simulink model "FaultFeeder"  (R2019a)
settings: Solver=ode1  StartTime=0.0  StopTime=2.5  FixedStep=Ts_Power  RelTol=1e-3
PostLoadFcn:
  | %% Init for wind PnO models - global system parameters
  | OVERRIDE_SSN_MEMORY_LIMIT=1;
  | Ts=50e-6;
  | % Ts=50e-10;
  | Ts_Power=Ts;
  | Ts_Control=2*Ts;
  | freq = 50;
  | Fnom=freq;
  | Vac=400e3;
InitFcn:
  | %% Init for wind PnO models - global system parameters
  | OVERRIDE_SSN_MEMORY_LIMIT=1;
  | Ts=50e-6;
  | % Ts=50e-10;
  | Ts_Power=Ts;
  | Ts_Control=2*Ts;
  | freq = 50;
  | Fnom=freq;
  | Vac=225e3;
values from neighbouring files (symbols this model uses):
  feeder_posCap = 0.2e-006    (= 2e-07)    [variable.m]
  feeder_posInd = 0.00040107    [variable.m]
  feeder_posR = 0.14    [variable.m]
  feeder_zeroCap = 0.08    [variable.m]
  feeder_zeroInd = 0.00120321    [variable.m]
  feeder_zeroR = 0.42    [variable.m]
  sub_posCap = 0.16e-006    (= 1.6e-07)    [variable.m]
  sub_posInd = 0.001400563    [variable.m]
  sub_posR = 0.036    [variable.m]
  sub_zeroCap = 0.053333e-006    (= 5.3333e-08)    [variable.m]
  sub_zeroInd = 0.00420169    [variable.m]
  sub_zeroR = 0.108    [variable.m]
  transfo_L1 = 0.05999374    [variable.m]
  transfo_L2 = 0.05999374    [variable.m]
  transfo_R1 = 0.000866667    [variable.m]
  transfo_R2 = 0.00086667    [variable.m]
undefined symbols (not defined in the file or in its folder): D1, D11, Delta, den, DiscIntNeverNeededParam, dx, find_system, gcbh, num, out_Buses, out_WindFarms, sps_rtmsupport
libraries: powerlib x196, simulink x96, powerlib_meascontrol x96, elements x52, eeSinusoidalMeasurement x49, simulink_extras x42, spsVIMeasurementModel x33, eePowerMeasurement x15
(part 22 of 24)

== system FaultFeeder/SM_WT1/Wind Type IV Detailed v2.1 - 4/Control/Measurement and Transformation/Discrete 3-phase PLL-Driven Positive-Sequence Active & Reactive Power/Discrete 3-phase PLL-Driven Positive-Sequence Fundamental Value2 ==
  note: Discrete 3-phase PLL-Driven Positive-Sequence Fundamental Value
  note: Pierre Giroux, Gilbert Sybille
      | Power System Simulation Laboratory
      | IREQ, Hydro-Quebc
  Freq : Inport
  w : Inport  Port=2  PortDimensions=1
  abc : Inport  Port=3  PortDimensions=3
  Cartesian to Polar : simulink_extras/Transformations/Cartesian to Polar
  Demux : Demux  Outputs=3
  Discrete Variable Frequency Mean value1 : Subsystem  mask(Discrete Variable-Frequency Mean Value){Finit=Finit, Fmin=Fmin, Vinit=Imag_Init, Ts=Ts}
      mask prompts: Finit "Initial frequency (Hz):"; Fmin "Minimum frequency (Hz):"; Vinit "Initial input (DC component):"; Ts "Sample time:"
      mask help:
      | This discrete block computes the mean value of the input signal (port In) over a running window of one cycle of a specified frequency (port Freq).
      |
      | For the first cycle of simulation (specified by the parameter "Initial frequency"), the output is held to the value of the  "Initial input" parameter.
      |
      | The value of the parameter "Minimum frequency" is used to determine the buffer size of the "Variable Transport Delay" block found inside this subsystem.
      mask init:
      | MaxDelay=1/Fmin+Ts;
      | power_initmask();
      settings: OpenFcn=power_openblockproxy();
  Discrete Variable Frequency Mean value2 : Subsystem  mask(Discrete Variable-Frequency Mean Value){Finit=Finit, Fmin=Fmin, Vinit=Real_Init, Ts=Ts}
      mask prompts: Finit "Initial frequency (Hz):"; Fmin "Minimum frequency (Hz):"; Vinit "Initial input (DC component):"; Ts "Sample time:"
      mask help:
      | This discrete block computes the mean value of the input signal (port In) over a running window of one cycle of a specified frequency (port Freq).
      |
      | For the first cycle of simulation (specified by the parameter "Initial frequency"), the output is held to the value of the  "Initial input" parameter.
      |
      | The value of the parameter "Minimum frequency" is used to determine the buffer size of the "Variable Transport Delay" block found inside this subsystem.
      mask init:
      | MaxDelay=1/Fmin+Ts;
      | power_initmask();
      settings: OpenFcn=power_openblockproxy();
  Rad->Deg. : Gain  Gain=180/pi  SaturateOnIntegerOverflow=on  OutDataTypeStr=Inherit: Same as input  ParamDataTypeStr=Inherit: Same as input
  Terminator : Terminator
  abc to dq0 : powerlib_meascontrol/Transformations/abc to dq0  Alignment=90 degrees behind phase A axis
  Mag : Outport  VectorParamsAs1DForOutWhenUnconnected=on
  Phase : Outport  Port=2  VectorParamsAs1DForOutWhenUnconnected=on
  wires:
  Cartesian to Polar/2 -> Rad->Deg./1
  Cartesian to Polar/1 -> Mag/1
  Demux/3 -> Terminator/1
  abc to dq0/1 -> Demux/1
  abc/1 -> abc to dq0/1
  Demux/1 -> Discrete Variable Frequency Mean value2/2(In)
  Demux/2 -> Discrete Variable Frequency Mean value1/2(In)
  Discrete Variable Frequency Mean value1/1(Mean) -> Cartesian to Polar/2  "Real"
  Rad->Deg./1 -> Phase/1
  Discrete Variable Frequency Mean value2/1(Mean) -> Cartesian to Polar/1  "Real"
  Freq/1 -> Discrete Variable Frequency Mean value1/1(Freq), Discrete Variable Frequency Mean value2/1(Freq)
  w/1 -> abc to dq0/2

== system FaultFeeder/SM_WT1/Wind Type IV Detailed v2.1 - 5/Control/Measurement and Transformation/Discrete 3-phase PLL-Driven Positive-Sequence Active & Reactive Power/Discrete 3-phase PLL-Driven Positive-Sequence Fundamental Value ==
  note: Pierre Giroux, Gilbert Sybille
      | Power System Simulation Laboratory
      | IREQ, Hydro-Quebc
  note: Discrete 3-phase PLL-Driven Positive-Sequence Fundamental Value
  Freq : Inport
  w : Inport  Port=2  PortDimensions=1
  abc : Inport  Port=3  PortDimensions=3
  Cartesian to Polar : simulink_extras/Transformations/Cartesian to Polar
  Demux : Demux  Outputs=3
  Discrete Variable Frequency Mean value1 : Subsystem  mask(Discrete Variable-Frequency Mean Value){Finit=Finit, Fmin=Fmin, Vinit=Imag_Init, Ts=Ts}
      mask prompts: Finit "Initial frequency (Hz):"; Fmin "Minimum frequency (Hz):"; Vinit "Initial input (DC component):"; Ts "Sample time:"
      mask help:
      | This discrete block computes the mean value of the input signal (port In) over a running window of one cycle of a specified frequency (port Freq).
      |
      | For the first cycle of simulation (specified by the parameter "Initial frequency"), the output is held to the value of the  "Initial input" parameter.
      |
      | The value of the parameter "Minimum frequency" is used to determine the buffer size of the "Variable Transport Delay" block found inside this subsystem.
      mask init:
      | MaxDelay=1/Fmin+Ts;
      | power_initmask();
      settings: OpenFcn=power_openblockproxy();
  Discrete Variable Frequency Mean value2 : Subsystem  mask(Discrete Variable-Frequency Mean Value){Finit=Finit, Fmin=Fmin, Vinit=Real_Init, Ts=Ts}
      mask prompts: Finit "Initial frequency (Hz):"; Fmin "Minimum frequency (Hz):"; Vinit "Initial input (DC component):"; Ts "Sample time:"
      mask help:
      | This discrete block computes the mean value of the input signal (port In) over a running window of one cycle of a specified frequency (port Freq).
      |
      | For the first cycle of simulation (specified by the parameter "Initial frequency"), the output is held to the value of the  "Initial input" parameter.
      |
      | The value of the parameter "Minimum frequency" is used to determine the buffer size of the "Variable Transport Delay" block found inside this subsystem.
      mask init:
      | MaxDelay=1/Fmin+Ts;
      | power_initmask();
      settings: OpenFcn=power_openblockproxy();
  Rad->Deg. : Gain  Gain=180/pi  SaturateOnIntegerOverflow=on  OutDataTypeStr=Inherit: Same as input  ParamDataTypeStr=Inherit: Same as input
  Terminator : Terminator
  abc to dq0 : powerlib_meascontrol/Transformations/abc to dq0  Alignment=90 degrees behind phase A axis
  Mag : Outport  VectorParamsAs1DForOutWhenUnconnected=on
  Phase : Outport  Port=2  VectorParamsAs1DForOutWhenUnconnected=on
  wires:
  w/1 -> abc to dq0/2
  Freq/1 -> Discrete Variable Frequency Mean value2/1(Freq), Discrete Variable Frequency Mean value1/1(Freq)
  Discrete Variable Frequency Mean value2/1(Mean) -> Cartesian to Polar/1  "Real"
  Rad->Deg./1 -> Phase/1
  Discrete Variable Frequency Mean value1/1(Mean) -> Cartesian to Polar/2  "Real"
  Demux/2 -> Discrete Variable Frequency Mean value1/2(In)
  Demux/1 -> Discrete Variable Frequency Mean value2/2(In)
  abc/1 -> abc to dq0/1
  abc to dq0/1 -> Demux/1
  Demux/3 -> Terminator/1
  Cartesian to Polar/1 -> Mag/1
  Cartesian to Polar/2 -> Rad->Deg./1

== system FaultFeeder/SM_WT1/Wind Type IV Detailed v2.1 - 5/Control/Measurement and Transformation/Discrete 3-phase PLL-Driven Positive-Sequence Active & Reactive Power/Discrete 3-phase PLL-Driven Positive-Sequence Fundamental Value2 ==
  note: Discrete 3-phase PLL-Driven Positive-Sequence Fundamental Value
  note: Pierre Giroux, Gilbert Sybille
      | Power System Simulation Laboratory
      | IREQ, Hydro-Quebc
  Freq : Inport
  w : Inport  Port=2  PortDimensions=1
  abc : Inport  Port=3  PortDimensions=3
  Cartesian to Polar : simulink_extras/Transformations/Cartesian to Polar
  Demux : Demux  Outputs=3
  Discrete Variable Frequency Mean value1 : Subsystem  mask(Discrete Variable-Frequency Mean Value){Finit=Finit, Fmin=Fmin, Vinit=Imag_Init, Ts=Ts}
      mask prompts: Finit "Initial frequency (Hz):"; Fmin "Minimum frequency (Hz):"; Vinit "Initial input (DC component):"; Ts "Sample time:"
      mask help:
      | This discrete block computes the mean value of the input signal (port In) over a running window of one cycle of a specified frequency (port Freq).
      |
      | For the first cycle of simulation (specified by the parameter "Initial frequency"), the output is held to the value of the  "Initial input" parameter.
      |
      | The value of the parameter "Minimum frequency" is used to determine the buffer size of the "Variable Transport Delay" block found inside this subsystem.
      mask init:
      | MaxDelay=1/Fmin+Ts;
      | power_initmask();
      settings: OpenFcn=power_openblockproxy();
  Discrete Variable Frequency Mean value2 : Subsystem  mask(Discrete Variable-Frequency Mean Value){Finit=Finit, Fmin=Fmin, Vinit=Real_Init, Ts=Ts}
      mask prompts: Finit "Initial frequency (Hz):"; Fmin "Minimum frequency (Hz):"; Vinit "Initial input (DC component):"; Ts "Sample time:"
      mask help:
      | This discrete block computes the mean value of the input signal (port In) over a running window of one cycle of a specified frequency (port Freq).
      |
      | For the first cycle of simulation (specified by the parameter "Initial frequency"), the output is held to the value of the  "Initial input" parameter.
      |
      | The value of the parameter "Minimum frequency" is used to determine the buffer size of the "Variable Transport Delay" block found inside this subsystem.
      mask init:
      | MaxDelay=1/Fmin+Ts;
      | power_initmask();
      settings: OpenFcn=power_openblockproxy();
  Rad->Deg. : Gain  Gain=180/pi  SaturateOnIntegerOverflow=on  OutDataTypeStr=Inherit: Same as input  ParamDataTypeStr=Inherit: Same as input
  Terminator : Terminator
  abc to dq0 : powerlib_meascontrol/Transformations/abc to dq0  Alignment=90 degrees behind phase A axis
  Mag : Outport  VectorParamsAs1DForOutWhenUnconnected=on
  Phase : Outport  Port=2  VectorParamsAs1DForOutWhenUnconnected=on
  wires:
  Cartesian to Polar/2 -> Rad->Deg./1
  Cartesian to Polar/1 -> Mag/1
  Demux/3 -> Terminator/1
  abc to dq0/1 -> Demux/1
  abc/1 -> abc to dq0/1
  Demux/1 -> Discrete Variable Frequency Mean value2/2(In)
  Demux/2 -> Discrete Variable Frequency Mean value1/2(In)
  Discrete Variable Frequency Mean value1/1(Mean) -> Cartesian to Polar/2  "Real"
  Rad->Deg./1 -> Phase/1
  Discrete Variable Frequency Mean value2/1(Mean) -> Cartesian to Polar/1  "Real"
  Freq/1 -> Discrete Variable Frequency Mean value1/1(Freq), Discrete Variable Frequency Mean value2/1(Freq)
  w/1 -> abc to dq0/2

== system FaultFeeder/SM_WT1/Wind Type IV Detailed v2.1 - 6/Control/Measurement and Transformation/Discrete 3-phase PLL-Driven Positive-Sequence Active & Reactive Power/Discrete 3-phase PLL-Driven Positive-Sequence Fundamental Value ==
  note: Pierre Giroux, Gilbert Sybille
      | Power System Simulation Laboratory
      | IREQ, Hydro-Quebc
  note: Discrete 3-phase PLL-Driven Positive-Sequence Fundamental Value
  Freq : Inport
  w : Inport  Port=2  PortDimensions=1
  abc : Inport  Port=3  PortDimensions=3
  Cartesian to Polar : simulink_extras/Transformations/Cartesian to Polar
  Demux : Demux  Outputs=3
  Discrete Variable Frequency Mean value1 : Subsystem  mask(Discrete Variable-Frequency Mean Value){Finit=Finit, Fmin=Fmin, Vinit=Imag_Init, Ts=Ts}
      mask prompts: Finit "Initial frequency (Hz):"; Fmin "Minimum frequency (Hz):"; Vinit "Initial input (DC component):"; Ts "Sample time:"
      mask help:
      | This discrete block computes the mean value of the input signal (port In) over a running window of one cycle of a specified frequency (port Freq).
      |
      | For the first cycle of simulation (specified by the parameter "Initial frequency"), the output is held to the value of the  "Initial input" parameter.
      |
      | The value of the parameter "Minimum frequency" is used to determine the buffer size of the "Variable Transport Delay" block found inside this subsystem.
      mask init:
      | MaxDelay=1/Fmin+Ts;
      | power_initmask();
      settings: OpenFcn=power_openblockproxy();
  Discrete Variable Frequency Mean value2 : Subsystem  mask(Discrete Variable-Frequency Mean Value){Finit=Finit, Fmin=Fmin, Vinit=Real_Init, Ts=Ts}
      mask prompts: Finit "Initial frequency (Hz):"; Fmin "Minimum frequency (Hz):"; Vinit "Initial input (DC component):"; Ts "Sample time:"
      mask help:
      | This discrete block computes the mean value of the input signal (port In) over a running window of one cycle of a specified frequency (port Freq).
      |
      | For the first cycle of simulation (specified by the parameter "Initial frequency"), the output is held to the value of the  "Initial input" parameter.
      |
      | The value of the parameter "Minimum frequency" is used to determine the buffer size of the "Variable Transport Delay" block found inside this subsystem.
      mask init:
      | MaxDelay=1/Fmin+Ts;
      | power_initmask();
      settings: OpenFcn=power_openblockproxy();
  Rad->Deg. : Gain  Gain=180/pi  SaturateOnIntegerOverflow=on  OutDataTypeStr=Inherit: Same as input  ParamDataTypeStr=Inherit: Same as input
  Terminator : Terminator
  abc to dq0 : powerlib_meascontrol/Transformations/abc to dq0  Alignment=90 degrees behind phase A axis
  Mag : Outport  VectorParamsAs1DForOutWhenUnconnected=on
  Phase : Outport  Port=2  VectorParamsAs1DForOutWhenUnconnected=on
  wires:
  w/1 -> abc to dq0/2
  Freq/1 -> Discrete Variable Frequency Mean value2/1(Freq), Discrete Variable Frequency Mean value1/1(Freq)
  Discrete Variable Frequency Mean value2/1(Mean) -> Cartesian to Polar/1  "Real"
  Rad->Deg./1 -> Phase/1
  Discrete Variable Frequency Mean value1/1(Mean) -> Cartesian to Polar/2  "Real"
  Demux/2 -> Discrete Variable Frequency Mean value1/2(In)
  Demux/1 -> Discrete Variable Frequency Mean value2/2(In)
  abc/1 -> abc to dq0/1
  abc to dq0/1 -> Demux/1
  Demux/3 -> Terminator/1
  Cartesian to Polar/1 -> Mag/1
  Cartesian to Polar/2 -> Rad->Deg./1

== system FaultFeeder/SM_WT1/Wind Type IV Detailed v2.1 - 6/Control/Measurement and Transformation/Discrete 3-phase PLL-Driven Positive-Sequence Active & Reactive Power/Discrete 3-phase PLL-Driven Positive-Sequence Fundamental Value2 ==
  note: Discrete 3-phase PLL-Driven Positive-Sequence Fundamental Value
  note: Pierre Giroux, Gilbert Sybille
      | Power System Simulation Laboratory
      | IREQ, Hydro-Quebc
  Freq : Inport
  w : Inport  Port=2  PortDimensions=1
  abc : Inport  Port=3  PortDimensions=3
  Cartesian to Polar : simulink_extras/Transformations/Cartesian to Polar
  Demux : Demux  Outputs=3
  Discrete Variable Frequency Mean value1 : Subsystem  mask(Discrete Variable-Frequency Mean Value){Finit=Finit, Fmin=Fmin, Vinit=Imag_Init, Ts=Ts}
      mask prompts: Finit "Initial frequency (Hz):"; Fmin "Minimum frequency (Hz):"; Vinit "Initial input (DC component):"; Ts "Sample time:"
      mask help:
      | This discrete block computes the mean value of the input signal (port In) over a running window of one cycle of a specified frequency (port Freq).
      |
      | For the first cycle of simulation (specified by the parameter "Initial frequency"), the output is held to the value of the  "Initial input" parameter.
      |
      | The value of the parameter "Minimum frequency" is used to determine the buffer size of the "Variable Transport Delay" block found inside this subsystem.
      mask init:
      | MaxDelay=1/Fmin+Ts;
      | power_initmask();
      settings: OpenFcn=power_openblockproxy();
  Discrete Variable Frequency Mean value2 : Subsystem  mask(Discrete Variable-Frequency Mean Value){Finit=Finit, Fmin=Fmin, Vinit=Real_Init, Ts=Ts}
      mask prompts: Finit "Initial frequency (Hz):"; Fmin "Minimum frequency (Hz):"; Vinit "Initial input (DC component):"; Ts "Sample time:"
      mask help:
      | This discrete block computes the mean value of the input signal (port In) over a running window of one cycle of a specified frequency (port Freq).
      |
      | For the first cycle of simulation (specified by the parameter "Initial frequency"), the output is held to the value of the  "Initial input" parameter.
      |
      | The value of the parameter "Minimum frequency" is used to determine the buffer size of the "Variable Transport Delay" block found inside this subsystem.
      mask init:
      | MaxDelay=1/Fmin+Ts;
      | power_initmask();
      settings: OpenFcn=power_openblockproxy();
  Rad->Deg. : Gain  Gain=180/pi  SaturateOnIntegerOverflow=on  OutDataTypeStr=Inherit: Same as input  ParamDataTypeStr=Inherit: Same as input
  Terminator : Terminator
  abc to dq0 : powerlib_meascontrol/Transformations/abc to dq0  Alignment=90 degrees behind phase A axis
  Mag : Outport  VectorParamsAs1DForOutWhenUnconnected=on
  Phase : Outport  Port=2  VectorParamsAs1DForOutWhenUnconnected=on
  wires:
  Cartesian to Polar/2 -> Rad->Deg./1
  Cartesian to Polar/1 -> Mag/1
  Demux/3 -> Terminator/1
  abc to dq0/1 -> Demux/1
  abc/1 -> abc to dq0/1
  Demux/1 -> Discrete Variable Frequency Mean value2/2(In)
  Demux/2 -> Discrete Variable Frequency Mean value1/2(In)
  Discrete Variable Frequency Mean value1/1(Mean) -> Cartesian to Polar/2  "Real"
  Rad->Deg./1 -> Phase/1
  Discrete Variable Frequency Mean value2/1(Mean) -> Cartesian to Polar/1  "Real"
  Freq/1 -> Discrete Variable Frequency Mean value1/1(Freq), Discrete Variable Frequency Mean value2/1(Freq)
  w/1 -> abc to dq0/2

== system FaultFeeder/SM_WT1/Wind Type IV Detailed v2.1 - 1/Control/Measurement and Transformation/Discrete 3-phase PLL-Driven Positive-Sequence Active & Reactive Power/Discrete 3-phase PLL-Driven Positive-Sequence Fundamental Value/Discrete Variable Frequency Mean value1 ==
  note: Variable frequency - Discrete Mean Value
  note: Pierre Giroux, Gilbert Sybille, Richard Gagnon
      | Power System Simulation Laboratory
      | IREQ, Hydro-Quebc
  Freq : Inport  PortDimensions=1
  In : Inport  Port=2  PortDimensions=1
  Correction subsystem : Subsystem
  Discrete Variable Transport Delay : Subsystem  mask(Discrete variable transport delay){MaxDelay=MaxDelay, InitialValue=0, Ts=Ts}
      mask prompts: MaxDelay "Maximum delay (s):"; InitialValue "Initial input:"; Ts "Sample time:"
      mask help:
      | Apply a delay to the first input (In) signal.
      | The second input (D) specifies the delay time.
  Gain : Gain  Gain=Ts  SaturateOnIntegerOverflow=on  OutDataTypeStr=Inherit: Same as input  ParamDataTypeStr=Inherit: Same as input
  Integ4 : DiscreteIntegrator  IntegratorMethod=Integration: Trapezoidal  SampleTime=Ts  ICPrevOutput=DiscIntNeverNeededParam  ICPrevScaledInput=DiscIntNeverNeededParam
  Number of samples per cycle : Fcn  Expr=1/u[1]/Ts
  Product : Product  SaturateOnIntegerOverflow=on  InputSameDT=on  OutDataTypeStr=Inherit: Same as first input
  Rounding Function : Rounding  Operator=ceil
  Step : Step  Time=1/Finit  SampleTime=Ts
  Sum5 : Sum  SaturateOnIntegerOverflow=on  InputSameDT=on  OutDataTypeStr=Inherit: Same as first input
  Sum7 : Sum  Inputs=-+  SaturateOnIntegerOverflow=on  InputSameDT=on  OutDataTypeStr=Inherit: Same as first input
  Switch : Switch  Threshold=0.5  InputSameDT=on
  To avoid division by zero : Saturate  UpperLimit=1e6  LowerLimit=1e-6
  Unit Delay : UnitDelay  InitialCondition=Vinit  SampleTime=Ts  HasFrameUpgradeWarning=on
  Mean : Outport  VectorParamsAs1DForOutWhenUnconnected=on
  wires:
  Step/1 -> Switch/2
  Correction subsystem/1(Out) -> Sum5/2
  To avoid division by zero/1 -> Number of samples per cycle/1  "Freq"
  Switch/1 -> Unit Delay/1, Mean/1
  Unit Delay/1 -> Switch/3
  Sum5/1 -> Switch/1
  Number of samples per cycle/1 -> Correction subsystem/1(N), Rounding Function/1
  Rounding Function/1 -> Correction subsystem/2(F), Gain/1
  Gain/1 -> Discrete Variable Transport Delay/2(D)  "Delay"
  Freq/1 -> To avoid division by zero/1, Product/2  "Freq"
  Integ4/1 -> Sum7/2, Discrete Variable Transport Delay/1(In)
  Sum7/1 -> Product/1
  Discrete Variable Transport Delay/1(Out) -> Sum7/1
  Product/1 -> Sum5/1  "Mean value"
  In/1 -> Correction subsystem/3(In), Integ4/1  "In"

== system FaultFeeder/SM_WT1/Wind Type IV Detailed v2.1 - 1/Control/Measurement and Transformation/Discrete 3-phase PLL-Driven Positive-Sequence Active & Reactive Power/Discrete 3-phase PLL-Driven Positive-Sequence Fundamental Value/Discrete Variable Frequency Mean value2 ==
  note: Pierre Giroux, Gilbert Sybille, Richard Gagnon
      | Power System Simulation Laboratory
      | IREQ, Hydro-Quebc
  note: Variable frequency - Discrete Mean Value
  Freq : Inport  PortDimensions=1
  In : Inport  Port=2  PortDimensions=1
  Correction subsystem : Subsystem
  Discrete Variable Transport Delay : Subsystem  mask(Discrete variable transport delay){MaxDelay=MaxDelay, InitialValue=0, Ts=Ts}
      mask prompts: MaxDelay "Maximum delay (s):"; InitialValue "Initial input:"; Ts "Sample time:"
      mask help:
      | Apply a delay to the first input (In) signal.
      | The second input (D) specifies the delay time.
  Gain : Gain  Gain=Ts  SaturateOnIntegerOverflow=on  OutDataTypeStr=Inherit: Same as input  ParamDataTypeStr=Inherit: Same as input
  Integ4 : DiscreteIntegrator  IntegratorMethod=Integration: Trapezoidal  SampleTime=Ts  ICPrevOutput=DiscIntNeverNeededParam  ICPrevScaledInput=DiscIntNeverNeededParam
  Number of samples per cycle : Fcn  Expr=1/u[1]/Ts
  Product : Product  SaturateOnIntegerOverflow=on  InputSameDT=on  OutDataTypeStr=Inherit: Same as first input
  Rounding Function : Rounding  Operator=ceil
  Step : Step  Time=1/Finit  SampleTime=Ts
  Sum5 : Sum  SaturateOnIntegerOverflow=on  InputSameDT=on  OutDataTypeStr=Inherit: Same as first input
  Sum7 : Sum  Inputs=-+  SaturateOnIntegerOverflow=on  InputSameDT=on  OutDataTypeStr=Inherit: Same as first input
  Switch : Switch  Threshold=0.5  InputSameDT=on
  To avoid division by zero : Saturate  UpperLimit=1e6  LowerLimit=1e-6
  Unit Delay : UnitDelay  InitialCondition=Vinit  SampleTime=Ts  HasFrameUpgradeWarning=on
  Mean : Outport  VectorParamsAs1DForOutWhenUnconnected=on
  wires:
  In/1 -> Integ4/1, Correction subsystem/3(In)  "In"
  Product/1 -> Sum5/1  "Mean value"
  Discrete Variable Transport Delay/1(Out) -> Sum7/1
  Sum7/1 -> Product/1
  Integ4/1 -> Discrete Variable Transport Delay/1(In), Sum7/2
  Freq/1 -> Product/2, To avoid division by zero/1  "Freq"
  Gain/1 -> Discrete Variable Transport Delay/2(D)  "Delay"
  Rounding Function/1 -> Gain/1, Correction subsystem/2(F)
  Number of samples per cycle/1 -> Rounding Function/1, Correction subsystem/1(N)
  Sum5/1 -> Switch/1
  Unit Delay/1 -> Switch/3
  Switch/1 -> Mean/1, Unit Delay/1
  To avoid division by zero/1 -> Number of samples per cycle/1  "Freq"
  Correction subsystem/1(Out) -> Sum5/2
  Step/1 -> Switch/2

== system FaultFeeder/SM_WT1/Wind Type IV Detailed v2.1 - 1/Control/Measurement and Transformation/Discrete 3-phase PLL-Driven Positive-Sequence Active & Reactive Power/Discrete 3-phase PLL-Driven Positive-Sequence Fundamental Value2/Discrete Variable Frequency Mean value1 ==
  note: Pierre Giroux, Gilbert Sybille, Richard Gagnon
      | Power System Simulation Laboratory
      | IREQ, Hydro-Quebc
  note: Variable frequency - Discrete Mean Value
  Freq : Inport  PortDimensions=1
  In : Inport  Port=2  PortDimensions=1
  Correction subsystem : Subsystem
  Discrete Variable Transport Delay : Subsystem  mask(Discrete variable transport delay){MaxDelay=MaxDelay, InitialValue=0, Ts=Ts}
      mask prompts: MaxDelay "Maximum delay (s):"; InitialValue "Initial input:"; Ts "Sample time:"
      mask help:
      | Apply a delay to the first input (In) signal.
      | The second input (D) specifies the delay time.
  Gain : Gain  Gain=Ts  SaturateOnIntegerOverflow=on  OutDataTypeStr=Inherit: Same as input  ParamDataTypeStr=Inherit: Same as input
  Integ4 : DiscreteIntegrator  IntegratorMethod=Integration: Trapezoidal  SampleTime=Ts  ICPrevOutput=DiscIntNeverNeededParam  ICPrevScaledInput=DiscIntNeverNeededParam
  Number of samples per cycle : Fcn  Expr=1/u[1]/Ts
  Product : Product  SaturateOnIntegerOverflow=on  InputSameDT=on  OutDataTypeStr=Inherit: Same as first input
  Rounding Function : Rounding  Operator=ceil
  Step : Step  Time=1/Finit  SampleTime=Ts
  Sum5 : Sum  SaturateOnIntegerOverflow=on  InputSameDT=on  OutDataTypeStr=Inherit: Same as first input
  Sum7 : Sum  Inputs=-+  SaturateOnIntegerOverflow=on  InputSameDT=on  OutDataTypeStr=Inherit: Same as first input
  Switch : Switch  Threshold=0.5  InputSameDT=on
  To avoid division by zero : Saturate  UpperLimit=1e6  LowerLimit=1e-6
  Unit Delay : UnitDelay  InitialCondition=Vinit  SampleTime=Ts  HasFrameUpgradeWarning=on
  Mean : Outport  VectorParamsAs1DForOutWhenUnconnected=on
  wires:
  In/1 -> Integ4/1, Correction subsystem/3(In)  "In"
  Product/1 -> Sum5/1  "Mean value"
  Discrete Variable Transport Delay/1(Out) -> Sum7/1
  Sum7/1 -> Product/1
  Integ4/1 -> Discrete Variable Transport Delay/1(In), Sum7/2
  Freq/1 -> Product/2, To avoid division by zero/1  "Freq"
  Gain/1 -> Discrete Variable Transport Delay/2(D)  "Delay"
  Rounding Function/1 -> Gain/1, Correction subsystem/2(F)
  Number of samples per cycle/1 -> Rounding Function/1, Correction subsystem/1(N)
  Sum5/1 -> Switch/1
  Unit Delay/1 -> Switch/3
  Switch/1 -> Mean/1, Unit Delay/1
  To avoid division by zero/1 -> Number of samples per cycle/1  "Freq"
  Correction subsystem/1(Out) -> Sum5/2
  Step/1 -> Switch/2

== system FaultFeeder/SM_WT1/Wind Type IV Detailed v2.1 - 1/Control/Measurement and Transformation/Discrete 3-phase PLL-Driven Positive-Sequence Active & Reactive Power/Discrete 3-phase PLL-Driven Positive-Sequence Fundamental Value2/Discrete Variable Frequency Mean value2 ==
  note: Variable frequency - Discrete Mean Value
  note: Pierre Giroux, Gilbert Sybille, Richard Gagnon
      | Power System Simulation Laboratory
      | IREQ, Hydro-Quebc
  Freq : Inport  PortDimensions=1
  In : Inport  Port=2  PortDimensions=1
  Correction subsystem : Subsystem
  Discrete Variable Transport Delay : Subsystem  mask(Discrete variable transport delay){MaxDelay=MaxDelay, InitialValue=0, Ts=Ts}
      mask prompts: MaxDelay "Maximum delay (s):"; InitialValue "Initial input:"; Ts "Sample time:"
      mask help:
      | Apply a delay to the first input (In) signal.
      | The second input (D) specifies the delay time.
  Gain : Gain  Gain=Ts  SaturateOnIntegerOverflow=on  OutDataTypeStr=Inherit: Same as input  ParamDataTypeStr=Inherit: Same as input
  Integ4 : DiscreteIntegrator  IntegratorMethod=Integration: Trapezoidal  SampleTime=Ts  ICPrevOutput=DiscIntNeverNeededParam  ICPrevScaledInput=DiscIntNeverNeededParam
  Number of samples per cycle : Fcn  Expr=1/u[1]/Ts
  Product : Product  SaturateOnIntegerOverflow=on  InputSameDT=on  OutDataTypeStr=Inherit: Same as first input
  Rounding Function : Rounding  Operator=ceil
  Step : Step  Time=1/Finit  SampleTime=Ts
  Sum5 : Sum  SaturateOnIntegerOverflow=on  InputSameDT=on  OutDataTypeStr=Inherit: Same as first input
  Sum7 : Sum  Inputs=-+  SaturateOnIntegerOverflow=on  InputSameDT=on  OutDataTypeStr=Inherit: Same as first input
  Switch : Switch  Threshold=0.5  InputSameDT=on
  To avoid division by zero : Saturate  UpperLimit=1e6  LowerLimit=1e-6
  Unit Delay : UnitDelay  InitialCondition=Vinit  SampleTime=Ts  HasFrameUpgradeWarning=on
  Mean : Outport  VectorParamsAs1DForOutWhenUnconnected=on
  wires:
  Step/1 -> Switch/2
  Correction subsystem/1(Out) -> Sum5/2
  To avoid division by zero/1 -> Number of samples per cycle/1  "Freq"
  Switch/1 -> Unit Delay/1, Mean/1
  Unit Delay/1 -> Switch/3
  Sum5/1 -> Switch/1
  Number of samples per cycle/1 -> Correction subsystem/1(N), Rounding Function/1
  Rounding Function/1 -> Correction subsystem/2(F), Gain/1
  Gain/1 -> Discrete Variable Transport Delay/2(D)  "Delay"
  Freq/1 -> To avoid division by zero/1, Product/2  "Freq"
  Integ4/1 -> Sum7/2, Discrete Variable Transport Delay/1(In)
  Sum7/1 -> Product/1
  Discrete Variable Transport Delay/1(Out) -> Sum7/1
  Product/1 -> Sum5/1  "Mean value"
  In/1 -> Correction subsystem/3(In), Integ4/1  "In"

== system FaultFeeder/SM_WT1/Wind Type IV Detailed v2.1 - 2/Control/Measurement and Transformation/Discrete 3-phase PLL-Driven Positive-Sequence Active & Reactive Power/Discrete 3-phase PLL-Driven Positive-Sequence Fundamental Value/Discrete Variable Frequency Mean value1 ==
  note: Pierre Giroux, Gilbert Sybille, Richard Gagnon
      | Power System Simulation Laboratory
      | IREQ, Hydro-Quebc
  note: Variable frequency - Discrete Mean Value
  Freq : Inport  PortDimensions=1
  In : Inport  Port=2  PortDimensions=1
  Correction subsystem : Subsystem
  Discrete Variable Transport Delay : Subsystem  mask(Discrete variable transport delay){MaxDelay=MaxDelay, InitialValue=0, Ts=Ts}
      mask prompts: MaxDelay "Maximum delay (s):"; InitialValue "Initial input:"; Ts "Sample time:"
      mask help:
      | Apply a delay to the first input (In) signal.
      | The second input (D) specifies the delay time.
  Gain : Gain  Gain=Ts  SaturateOnIntegerOverflow=on  OutDataTypeStr=Inherit: Same as input  ParamDataTypeStr=Inherit: Same as input
  Integ4 : DiscreteIntegrator  IntegratorMethod=Integration: Trapezoidal  SampleTime=Ts  ICPrevOutput=DiscIntNeverNeededParam  ICPrevScaledInput=DiscIntNeverNeededParam
  Number of samples per cycle : Fcn  Expr=1/u[1]/Ts
  Product : Product  SaturateOnIntegerOverflow=on  InputSameDT=on  OutDataTypeStr=Inherit: Same as first input
  Rounding Function : Rounding  Operator=ceil
  Step : Step  Time=1/Finit  SampleTime=Ts
  Sum5 : Sum  SaturateOnIntegerOverflow=on  InputSameDT=on  OutDataTypeStr=Inherit: Same as first input
  Sum7 : Sum  Inputs=-+  SaturateOnIntegerOverflow=on  InputSameDT=on  OutDataTypeStr=Inherit: Same as first input
  Switch : Switch  Threshold=0.5  InputSameDT=on
  To avoid division by zero : Saturate  UpperLimit=1e6  LowerLimit=1e-6
  Unit Delay : UnitDelay  InitialCondition=Vinit  SampleTime=Ts  HasFrameUpgradeWarning=on
  Mean : Outport  VectorParamsAs1DForOutWhenUnconnected=on
  wires:
  In/1 -> Integ4/1, Correction subsystem/3(In)  "In"
  Product/1 -> Sum5/1  "Mean value"
  Discrete Variable Transport Delay/1(Out) -> Sum7/1
  Sum7/1 -> Product/1
  Integ4/1 -> Discrete Variable Transport Delay/1(In), Sum7/2
  Freq/1 -> Product/2, To avoid division by zero/1  "Freq"
  Gain/1 -> Discrete Variable Transport Delay/2(D)  "Delay"
  Rounding Function/1 -> Gain/1, Correction subsystem/2(F)
  Number of samples per cycle/1 -> Rounding Function/1, Correction subsystem/1(N)
  Sum5/1 -> Switch/1
  Unit Delay/1 -> Switch/3
  Switch/1 -> Mean/1, Unit Delay/1
  To avoid division by zero/1 -> Number of samples per cycle/1  "Freq"
  Correction subsystem/1(Out) -> Sum5/2
  Step/1 -> Switch/2

== system FaultFeeder/SM_WT1/Wind Type IV Detailed v2.1 - 2/Control/Measurement and Transformation/Discrete 3-phase PLL-Driven Positive-Sequence Active & Reactive Power/Discrete 3-phase PLL-Driven Positive-Sequence Fundamental Value/Discrete Variable Frequency Mean value2 ==
  note: Variable frequency - Discrete Mean Value
  note: Pierre Giroux, Gilbert Sybille, Richard Gagnon
      | Power System Simulation Laboratory
      | IREQ, Hydro-Quebc
  Freq : Inport  PortDimensions=1
  In : Inport  Port=2  PortDimensions=1
  Correction subsystem : Subsystem
  Discrete Variable Transport Delay : Subsystem  mask(Discrete variable transport delay){MaxDelay=MaxDelay, InitialValue=0, Ts=Ts}
      mask prompts: MaxDelay "Maximum delay (s):"; InitialValue "Initial input:"; Ts "Sample time:"
      mask help:
      | Apply a delay to the first input (In) signal.
      | The second input (D) specifies the delay time.
  Gain : Gain  Gain=Ts  SaturateOnIntegerOverflow=on  OutDataTypeStr=Inherit: Same as input  ParamDataTypeStr=Inherit: Same as input
  Integ4 : DiscreteIntegrator  IntegratorMethod=Integration: Trapezoidal  SampleTime=Ts  ICPrevOutput=DiscIntNeverNeededParam  ICPrevScaledInput=DiscIntNeverNeededParam
  Number of samples per cycle : Fcn  Expr=1/u[1]/Ts
  Product : Product  SaturateOnIntegerOverflow=on  InputSameDT=on  OutDataTypeStr=Inherit: Same as first input
  Rounding Function : Rounding  Operator=ceil
  Step : Step  Time=1/Finit  SampleTime=Ts
  Sum5 : Sum  SaturateOnIntegerOverflow=on  InputSameDT=on  OutDataTypeStr=Inherit: Same as first input
  Sum7 : Sum  Inputs=-+  SaturateOnIntegerOverflow=on  InputSameDT=on  OutDataTypeStr=Inherit: Same as first input
  Switch : Switch  Threshold=0.5  InputSameDT=on
  To avoid division by zero : Saturate  UpperLimit=1e6  LowerLimit=1e-6
  Unit Delay : UnitDelay  InitialCondition=Vinit  SampleTime=Ts  HasFrameUpgradeWarning=on
  Mean : Outport  VectorParamsAs1DForOutWhenUnconnected=on
  wires:
  Step/1 -> Switch/2
  Correction subsystem/1(Out) -> Sum5/2
  To avoid division by zero/1 -> Number of samples per cycle/1  "Freq"
  Switch/1 -> Unit Delay/1, Mean/1
  Unit Delay/1 -> Switch/3
  Sum5/1 -> Switch/1
  Number of samples per cycle/1 -> Correction subsystem/1(N), Rounding Function/1
  Rounding Function/1 -> Correction subsystem/2(F), Gain/1
  Gain/1 -> Discrete Variable Transport Delay/2(D)  "Delay"
  Freq/1 -> To avoid division by zero/1, Product/2  "Freq"
  Integ4/1 -> Sum7/2, Discrete Variable Transport Delay/1(In)
  Sum7/1 -> Product/1
  Discrete Variable Transport Delay/1(Out) -> Sum7/1
  Product/1 -> Sum5/1  "Mean value"
  In/1 -> Correction subsystem/3(In), Integ4/1  "In"

== system FaultFeeder/SM_WT1/Wind Type IV Detailed v2.1 - 2/Control/Measurement and Transformation/Discrete 3-phase PLL-Driven Positive-Sequence Active & Reactive Power/Discrete 3-phase PLL-Driven Positive-Sequence Fundamental Value2/Discrete Variable Frequency Mean value1 ==
  note: Variable frequency - Discrete Mean Value
  note: Pierre Giroux, Gilbert Sybille, Richard Gagnon
      | Power System Simulation Laboratory
      | IREQ, Hydro-Quebc
  Freq : Inport  PortDimensions=1
  In : Inport  Port=2  PortDimensions=1
  Correction subsystem : Subsystem
  Discrete Variable Transport Delay : Subsystem  mask(Discrete variable transport delay){MaxDelay=MaxDelay, InitialValue=0, Ts=Ts}
      mask prompts: MaxDelay "Maximum delay (s):"; InitialValue "Initial input:"; Ts "Sample time:"
      mask help:
      | Apply a delay to the first input (In) signal.
      | The second input (D) specifies the delay time.
  Gain : Gain  Gain=Ts  SaturateOnIntegerOverflow=on  OutDataTypeStr=Inherit: Same as input  ParamDataTypeStr=Inherit: Same as input
  Integ4 : DiscreteIntegrator  IntegratorMethod=Integration: Trapezoidal  SampleTime=Ts  ICPrevOutput=DiscIntNeverNeededParam  ICPrevScaledInput=DiscIntNeverNeededParam
  Number of samples per cycle : Fcn  Expr=1/u[1]/Ts
  Product : Product  SaturateOnIntegerOverflow=on  InputSameDT=on  OutDataTypeStr=Inherit: Same as first input
  Rounding Function : Rounding  Operator=ceil
  Step : Step  Time=1/Finit  SampleTime=Ts
  Sum5 : Sum  SaturateOnIntegerOverflow=on  InputSameDT=on  OutDataTypeStr=Inherit: Same as first input
  Sum7 : Sum  Inputs=-+  SaturateOnIntegerOverflow=on  InputSameDT=on  OutDataTypeStr=Inherit: Same as first input
  Switch : Switch  Threshold=0.5  InputSameDT=on
  To avoid division by zero : Saturate  UpperLimit=1e6  LowerLimit=1e-6
  Unit Delay : UnitDelay  InitialCondition=Vinit  SampleTime=Ts  HasFrameUpgradeWarning=on
  Mean : Outport  VectorParamsAs1DForOutWhenUnconnected=on
  wires:
  Step/1 -> Switch/2
  Correction subsystem/1(Out) -> Sum5/2
  To avoid division by zero/1 -> Number of samples per cycle/1  "Freq"
  Switch/1 -> Unit Delay/1, Mean/1
  Unit Delay/1 -> Switch/3
  Sum5/1 -> Switch/1
  Number of samples per cycle/1 -> Correction subsystem/1(N), Rounding Function/1
  Rounding Function/1 -> Correction subsystem/2(F), Gain/1
  Gain/1 -> Discrete Variable Transport Delay/2(D)  "Delay"
  Freq/1 -> To avoid division by zero/1, Product/2  "Freq"
  Integ4/1 -> Sum7/2, Discrete Variable Transport Delay/1(In)
  Sum7/1 -> Product/1
  Discrete Variable Transport Delay/1(Out) -> Sum7/1
  Product/1 -> Sum5/1  "Mean value"
  In/1 -> Correction subsystem/3(In), Integ4/1  "In"

== system FaultFeeder/SM_WT1/Wind Type IV Detailed v2.1 - 2/Control/Measurement and Transformation/Discrete 3-phase PLL-Driven Positive-Sequence Active & Reactive Power/Discrete 3-phase PLL-Driven Positive-Sequence Fundamental Value2/Discrete Variable Frequency Mean value2 ==
  note: Pierre Giroux, Gilbert Sybille, Richard Gagnon
      | Power System Simulation Laboratory
      | IREQ, Hydro-Quebc
  note: Variable frequency - Discrete Mean Value
  Freq : Inport  PortDimensions=1
  In : Inport  Port=2  PortDimensions=1
  Correction subsystem : Subsystem
  Discrete Variable Transport Delay : Subsystem  mask(Discrete variable transport delay){MaxDelay=MaxDelay, InitialValue=0, Ts=Ts}
      mask prompts: MaxDelay "Maximum delay (s):"; InitialValue "Initial input:"; Ts "Sample time:"
      mask help:
      | Apply a delay to the first input (In) signal.
      | The second input (D) specifies the delay time.
  Gain : Gain  Gain=Ts  SaturateOnIntegerOverflow=on  OutDataTypeStr=Inherit: Same as input  ParamDataTypeStr=Inherit: Same as input
  Integ4 : DiscreteIntegrator  IntegratorMethod=Integration: Trapezoidal  SampleTime=Ts  ICPrevOutput=DiscIntNeverNeededParam  ICPrevScaledInput=DiscIntNeverNeededParam
  Number of samples per cycle : Fcn  Expr=1/u[1]/Ts
  Product : Product  SaturateOnIntegerOverflow=on  InputSameDT=on  OutDataTypeStr=Inherit: Same as first input
  Rounding Function : Rounding  Operator=ceil
  Step : Step  Time=1/Finit  SampleTime=Ts
  Sum5 : Sum  SaturateOnIntegerOverflow=on  InputSameDT=on  OutDataTypeStr=Inherit: Same as first input
  Sum7 : Sum  Inputs=-+  SaturateOnIntegerOverflow=on  InputSameDT=on  OutDataTypeStr=Inherit: Same as first input
  Switch : Switch  Threshold=0.5  InputSameDT=on
  To avoid division by zero : Saturate  UpperLimit=1e6  LowerLimit=1e-6
  Unit Delay : UnitDelay  InitialCondition=Vinit  SampleTime=Ts  HasFrameUpgradeWarning=on
  Mean : Outport  VectorParamsAs1DForOutWhenUnconnected=on
  wires:
  In/1 -> Integ4/1, Correction subsystem/3(In)  "In"
  Product/1 -> Sum5/1  "Mean value"
  Discrete Variable Transport Delay/1(Out) -> Sum7/1
  Sum7/1 -> Product/1
  Integ4/1 -> Discrete Variable Transport Delay/1(In), Sum7/2
  Freq/1 -> Product/2, To avoid division by zero/1  "Freq"
  Gain/1 -> Discrete Variable Transport Delay/2(D)  "Delay"
  Rounding Function/1 -> Gain/1, Correction subsystem/2(F)
  Number of samples per cycle/1 -> Rounding Function/1, Correction subsystem/1(N)
  Sum5/1 -> Switch/1
  Unit Delay/1 -> Switch/3
  Switch/1 -> Mean/1, Unit Delay/1
  To avoid division by zero/1 -> Number of samples per cycle/1  "Freq"
  Correction subsystem/1(Out) -> Sum5/2
  Step/1 -> Switch/2

== system FaultFeeder/SM_WT1/Wind Type IV Detailed v2.1 - 3/Control/Measurement and Transformation/Discrete 3-phase PLL-Driven Positive-Sequence Active & Reactive Power/Discrete 3-phase PLL-Driven Positive-Sequence Fundamental Value/Discrete Variable Frequency Mean value1 ==
  note: Pierre Giroux, Gilbert Sybille, Richard Gagnon
      | Power System Simulation Laboratory
      | IREQ, Hydro-Quebc
  note: Variable frequency - Discrete Mean Value
  Freq : Inport  PortDimensions=1
  In : Inport  Port=2  PortDimensions=1
  Correction subsystem : Subsystem
  Discrete Variable Transport Delay : Subsystem  mask(Discrete variable transport delay){MaxDelay=MaxDelay, InitialValue=0, Ts=Ts}
      mask prompts: MaxDelay "Maximum delay (s):"; InitialValue "Initial input:"; Ts "Sample time:"
      mask help:
      | Apply a delay to the first input (In) signal.
      | The second input (D) specifies the delay time.
  Gain : Gain  Gain=Ts  SaturateOnIntegerOverflow=on  OutDataTypeStr=Inherit: Same as input  ParamDataTypeStr=Inherit: Same as input
  Integ4 : DiscreteIntegrator  IntegratorMethod=Integration: Trapezoidal  SampleTime=Ts  ICPrevOutput=DiscIntNeverNeededParam  ICPrevScaledInput=DiscIntNeverNeededParam
  Number of samples per cycle : Fcn  Expr=1/u[1]/Ts
  Product : Product  SaturateOnIntegerOverflow=on  InputSameDT=on  OutDataTypeStr=Inherit: Same as first input
  Rounding Function : Rounding  Operator=ceil
  Step : Step  Time=1/Finit  SampleTime=Ts
  Sum5 : Sum  SaturateOnIntegerOverflow=on  InputSameDT=on  OutDataTypeStr=Inherit: Same as first input
  Sum7 : Sum  Inputs=-+  SaturateOnIntegerOverflow=on  InputSameDT=on  OutDataTypeStr=Inherit: Same as first input
  Switch : Switch  Threshold=0.5  InputSameDT=on
  To avoid division by zero : Saturate  UpperLimit=1e6  LowerLimit=1e-6
  Unit Delay : UnitDelay  InitialCondition=Vinit  SampleTime=Ts  HasFrameUpgradeWarning=on
  Mean : Outport  VectorParamsAs1DForOutWhenUnconnected=on
  wires:
  In/1 -> Integ4/1, Correction subsystem/3(In)  "In"
  Product/1 -> Sum5/1  "Mean value"
  Discrete Variable Transport Delay/1(Out) -> Sum7/1
  Sum7/1 -> Product/1
  Integ4/1 -> Discrete Variable Transport Delay/1(In), Sum7/2
  Freq/1 -> Product/2, To avoid division by zero/1  "Freq"
  Gain/1 -> Discrete Variable Transport Delay/2(D)  "Delay"
  Rounding Function/1 -> Gain/1, Correction subsystem/2(F)
  Number of samples per cycle/1 -> Rounding Function/1, Correction subsystem/1(N)
  Sum5/1 -> Switch/1
  Unit Delay/1 -> Switch/3
  Switch/1 -> Mean/1, Unit Delay/1
  To avoid division by zero/1 -> Number of samples per cycle/1  "Freq"
  Correction subsystem/1(Out) -> Sum5/2
  Step/1 -> Switch/2

== system FaultFeeder/SM_WT1/Wind Type IV Detailed v2.1 - 3/Control/Measurement and Transformation/Discrete 3-phase PLL-Driven Positive-Sequence Active & Reactive Power/Discrete 3-phase PLL-Driven Positive-Sequence Fundamental Value/Discrete Variable Frequency Mean value2 ==
  note: Variable frequency - Discrete Mean Value
  note: Pierre Giroux, Gilbert Sybille, Richard Gagnon
      | Power System Simulation Laboratory
      | IREQ, Hydro-Quebc
  Freq : Inport  PortDimensions=1
  In : Inport  Port=2  PortDimensions=1
  Correction subsystem : Subsystem
  Discrete Variable Transport Delay : Subsystem  mask(Discrete variable transport delay){MaxDelay=MaxDelay, InitialValue=0, Ts=Ts}
      mask prompts: MaxDelay "Maximum delay (s):"; InitialValue "Initial input:"; Ts "Sample time:"
      mask help:
      | Apply a delay to the first input (In) signal.
      | The second input (D) specifies the delay time.
  Gain : Gain  Gain=Ts  SaturateOnIntegerOverflow=on  OutDataTypeStr=Inherit: Same as input  ParamDataTypeStr=Inherit: Same as input
  Integ4 : DiscreteIntegrator  IntegratorMethod=Integration: Trapezoidal  SampleTime=Ts  ICPrevOutput=DiscIntNeverNeededParam  ICPrevScaledInput=DiscIntNeverNeededParam
  Number of samples per cycle : Fcn  Expr=1/u[1]/Ts
  Product : Product  SaturateOnIntegerOverflow=on  InputSameDT=on  OutDataTypeStr=Inherit: Same as first input
  Rounding Function : Rounding  Operator=ceil
  Step : Step  Time=1/Finit  SampleTime=Ts
  Sum5 : Sum  SaturateOnIntegerOverflow=on  InputSameDT=on  OutDataTypeStr=Inherit: Same as first input
  Sum7 : Sum  Inputs=-+  SaturateOnIntegerOverflow=on  InputSameDT=on  OutDataTypeStr=Inherit: Same as first input
  Switch : Switch  Threshold=0.5  InputSameDT=on
  To avoid division by zero : Saturate  UpperLimit=1e6  LowerLimit=1e-6
  Unit Delay : UnitDelay  InitialCondition=Vinit  SampleTime=Ts  HasFrameUpgradeWarning=on
  Mean : Outport  VectorParamsAs1DForOutWhenUnconnected=on
  wires:
  Step/1 -> Switch/2
  Correction subsystem/1(Out) -> Sum5/2
  To avoid division by zero/1 -> Number of samples per cycle/1  "Freq"
  Switch/1 -> Unit Delay/1, Mean/1
  Unit Delay/1 -> Switch/3
  Sum5/1 -> Switch/1
  Number of samples per cycle/1 -> Correction subsystem/1(N), Rounding Function/1
  Rounding Function/1 -> Correction subsystem/2(F), Gain/1
  Gain/1 -> Discrete Variable Transport Delay/2(D)  "Delay"
  Freq/1 -> To avoid division by zero/1, Product/2  "Freq"
  Integ4/1 -> Sum7/2, Discrete Variable Transport Delay/1(In)
  Sum7/1 -> Product/1
  Discrete Variable Transport Delay/1(Out) -> Sum7/1
  Product/1 -> Sum5/1  "Mean value"
  In/1 -> Correction subsystem/3(In), Integ4/1  "In"

== system FaultFeeder/SM_WT1/Wind Type IV Detailed v2.1 - 3/Control/Measurement and Transformation/Discrete 3-phase PLL-Driven Positive-Sequence Active & Reactive Power/Discrete 3-phase PLL-Driven Positive-Sequence Fundamental Value2/Discrete Variable Frequency Mean value1 ==
  note: Variable frequency - Discrete Mean Value
  note: Pierre Giroux, Gilbert Sybille, Richard Gagnon
      | Power System Simulation Laboratory
      | IREQ, Hydro-Quebc
  Freq : Inport  PortDimensions=1
  In : Inport  Port=2  PortDimensions=1
  Correction subsystem : Subsystem
  Discrete Variable Transport Delay : Subsystem  mask(Discrete variable transport delay){MaxDelay=MaxDelay, InitialValue=0, Ts=Ts}
      mask prompts: MaxDelay "Maximum delay (s):"; InitialValue "Initial input:"; Ts "Sample time:"
      mask help:
      | Apply a delay to the first input (In) signal.
      | The second input (D) specifies the delay time.
  Gain : Gain  Gain=Ts  SaturateOnIntegerOverflow=on  OutDataTypeStr=Inherit: Same as input  ParamDataTypeStr=Inherit: Same as input
  Integ4 : DiscreteIntegrator  IntegratorMethod=Integration: Trapezoidal  SampleTime=Ts  ICPrevOutput=DiscIntNeverNeededParam  ICPrevScaledInput=DiscIntNeverNeededParam
  Number of samples per cycle : Fcn  Expr=1/u[1]/Ts
  Product : Product  SaturateOnIntegerOverflow=on  InputSameDT=on  OutDataTypeStr=Inherit: Same as first input
  Rounding Function : Rounding  Operator=ceil
  Step : Step  Time=1/Finit  SampleTime=Ts
  Sum5 : Sum  SaturateOnIntegerOverflow=on  InputSameDT=on  OutDataTypeStr=Inherit: Same as first input
  Sum7 : Sum  Inputs=-+  SaturateOnIntegerOverflow=on  InputSameDT=on  OutDataTypeStr=Inherit: Same as first input
  Switch : Switch  Threshold=0.5  InputSameDT=on
  To avoid division by zero : Saturate  UpperLimit=1e6  LowerLimit=1e-6
  Unit Delay : UnitDelay  InitialCondition=Vinit  SampleTime=Ts  HasFrameUpgradeWarning=on
  Mean : Outport  VectorParamsAs1DForOutWhenUnconnected=on
  wires:
  Step/1 -> Switch/2
  Correction subsystem/1(Out) -> Sum5/2
  To avoid division by zero/1 -> Number of samples per cycle/1  "Freq"
  Switch/1 -> Unit Delay/1, Mean/1
  Unit Delay/1 -> Switch/3
  Sum5/1 -> Switch/1
  Number of samples per cycle/1 -> Correction subsystem/1(N), Rounding Function/1
  Rounding Function/1 -> Correction subsystem/2(F), Gain/1
  Gain/1 -> Discrete Variable Transport Delay/2(D)  "Delay"
  Freq/1 -> To avoid division by zero/1, Product/2  "Freq"
  Integ4/1 -> Sum7/2, Discrete Variable Transport Delay/1(In)
  Sum7/1 -> Product/1
  Discrete Variable Transport Delay/1(Out) -> Sum7/1
  Product/1 -> Sum5/1  "Mean value"
  In/1 -> Correction subsystem/3(In), Integ4/1  "In"
